simulink model "AMCLIB_BemfObsrvDQ_BAM"  (Simulink 9.3)
settings: Solver=VariableStepAuto  StartTime=0.0  StopTime=10.0  RelTol=1e-3
settings Model: Creator=nxa18952  LastModifiedBy=nxa18952
settings DataIOCC: SaveFormat=Dataset  SignalLoggingSaveFormat=Dataset  ReturnWorkspaceOutputs=on
settings OptimizationCC: LifeSpan=auto
settings DebuggingCC: UnderspecifiedInitializationDetection=Simplified  MergeDetectMultiDrivingBlocksExec=error  FcnCallInpInsideContextMsg=error  SFUnexpectedBacktrackingDiag=error  SFNoUnconditionalDefaultTransitionDiag=error  SFExecutionAtInitializationDiag=warning  ArithmeticOperatorsInVariantConditions=error
settings HardwareCC: ProdBitPerPointer=64  ProdBitPerSizeT=64  ProdBitPerPtrDiffT=64  ProdLargestAtomicFloat=Float  ProdIntDivRoundTo=Zero  ProdEndianess=LittleEndian  ProdWordSize=64  ProdHWDeviceType=Intel->x86-64 (Windows64)
settings ModelReferenceCC: PropagateSignalLabelsOutOfModel=on
settings SFSimCC: SimUseLocalCustomCode=on
settings RTWCC: RTWUseLocalCustomCode=on
settings CodeAppCC: StateflowObjectComments=off
settings GRTTargetCC: TargetLangStandard=C99 (ISO)  CombineOutputUpdateFcns=on  GRTInterface=off
settings ConfigComp: CovMetricSettings=dwe  CovHtmlReporting=off  CovSaveCumulativeToWorkspaceVar=off  CovSaveSingleToWorkspaceVar=off  CovExternalEMLEnable=on

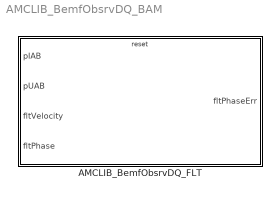
== system AMCLIB_BemfObsrvDQ_BAM ==
  AMCLIB_BemfObsrvDQ_FLT : Subsystem  TreatAsAtomicUnit=on  mask(AMCLIB_BemfObsrvDQ_FLT){showStates=Hide (faster execution), resetStatesEnable=Pre-set according to the first set of inputs after reset, fltIGain=0, fltUGain=0, fltWIGain=0, fltEGain=0, fltCC1sc_D=0, fltCC2sc_D=0, fltUpperLimit_D=0, fltLowerLimit_D=0, fltCC1sc_Q=0, fltCC2sc_Q=0, fltUpperLimit_Q=0, fltLowerLimit_Q=0}
      mask prompts: showStates "Show internal states"; resetStatesEnable "Internal state after reset"; fltIGain "fltIGain (RL circuit constant)"; fltUGain "fltUGain (Voltage cross-coupling constant)"; fltWIGain "fltWIGain (Angular velocity cross-coupling constant)"; fltEGain "fltEGain (Back-EMF cross-coupling constant)"; fltCC1sc_D "fltCC1sc_D (CC1 coefficient of the D-axis PI controller)"; fltCC2sc_D "fltCC2sc_D (CC2 coefficient of the D-axis PI controller)"; fltUpperLimit_D "fltUpperLimit_D (Upper Limit of the D-axis PI controller)"; fltLowerLimit_D "fltLowerLimit_D (Lower Limit of the D-axis PI controller)"; fltCC1sc_Q "fltCC1sc_Q (CC1 coefficient of the Q-axis PI controller)"; fltCC2sc_Q "fltCC2sc_Q (CC2 coefficient of the Q-axis PI controller)"; fltUpperLimit_Q "fltUpperLimit_Q (Upper Limit of the Q-axis PI controller)"; fltLowerLimit_Q "fltLowerLimit_Q (Lower Limit of the Q-axis PI controller)"
      mask help: PMSM back-EMF observer DQ in single precision floating-point implementation. This block supports re-initialization of the internal state during simulation. If the block is reset, the observer will align with the motor's position and speed measured in the next time step. This allows seamless on-the-fly transition to the closed-loop control. Refer to the AMMCLIB User's Guide for further details.
      mask init:
      | if ~evalin('base','exist(''tS8'',''var'')')
      |   if (2 ~= exist('SWLIBS_Typedefs.mat','file'))
      |       error('File SWLIBS_Typedefs.mat is not on the Matlab path. Please add the AMMCLIB "bam" folder in the Matlab Search Path.');
      |   else
      |       evalin('base', 'load(''SWLIBS_Typedefs.mat'')');
      |   end
      | end
      | if showStates == 1
      |     % hidden state variables
      |     if strcmp(get_param([gcb '/fltIGain'], 'BlockType'), 'Inport')
      |         posblk = get_param(gcb, 'Position');
      | 
      |         pos = get_param(    [gcb, '/fltIGain'], 'Position');
      |         orient = get_param( [gcb, '/fltIGain'], 'Orientation');
      |         delete_block(       [gcb, '/fltIGain']);
      |         add_block('built-in/Ground', [gcb, '/fltIGain'], 'Position', pos, 'Orientation', orient);
      | 
      |         pos = get_param(    [gcb, '/fltUGain'], 'Position');
      |         orient = get_param( [gcb, '/fltUGain'], 'Orientation');
      |         delete_block(       [gcb, '/fltUGain']);
      |         add_block('built-in/Ground', [gcb, '/fltUGain'], 'Position', pos, 'Orientation', orient);
      | 
      |         pos = get_param(    [gcb, '/fltWIGain'], 'Position');
      |         orient = get_param( [gcb, '/fltWIGain'], 'Orientation');
      |         delete_block(       [gcb, '/fltWIGain']);
      |         add_block('built-in/Ground', [gcb, '/fltWIGain'], 'Position', pos, 'Orientation', orient);
      | 
      |         pos = get_param(    [gcb, '/fltEGain'], 'Position');
      |         orient = get_param( [gcb, '/fltEGain'], 'Orientation');
      |         delete_block(       [gcb, '/fltEGain']);
      |         add_block('built-in/Ground', [gcb, '/fltEGain'], 'Position', pos, 'Orientation', orient);
      | 
      |         pos = get_param(    [gcb, '/fltCC1sc_D'], 'Position');
      |         orient = get_param( [gcb, '/fltCC1sc_D'], 'Orientation');
      |         delete_block(       [gcb, '/fltCC1sc_D']);
      |         add_block('built-in/Ground', [gcb, '/fltCC1sc_D'], 'Position', pos, 'Orientation', orient);
      | 
      |         pos = get_param(    [gcb, '/fltCC2sc_D'], 'Position');
      |         orient = get_param( [gcb, '/fltCC2sc_D'], 'Orientation');
      |         delete_block(       [gcb, '/fltCC2sc_D']);
      |         add_block('built-in/Ground', [gcb, '/fltCC2sc_D'], 'Position', pos, 'Orientation', orient);
      | 
      |         pos = get_param(    [gcb, '/fltUpperLimit_D'], 'Position');
      |         orient = get_param( [gcb, '/fltUpperLimit_D'], 'Orientation');
      |         delete_block(       [gcb, '/fltUpperLimit_D']);
      |         add_block('built-in/Ground', [gcb, '/fltUpperLimit_D'], 'Position', pos, 'Orientation', orient);
      | 
      |         pos = get_param(    [gcb, '/fltLowerLimit_D'], 'Position');
      |         orient = get_param( [gcb, '/fltLowerLimit_D'], 'Orientation');
      |         delete_block(       [gcb, '/fltLowerLimit_D']);
      |         add_block('built-in/Ground', [gcb, '/fltLowerLimit_D'], 'Position', pos, 'Orientation', orient);
      | 
      |         pos = get_param(    [gcb, '/fltCC1sc_Q'], 'Position');
      |         orient = get_param( [gcb, '/fltCC1sc_Q'], 'Orientation');
      |         delete_block(       [gcb, '/fltCC1sc_Q']);
      |         add_block('built-in/Ground', [gcb, '/fltCC1sc_Q'], 'Position', pos, 'Orientation', orient);
      | 
      |         pos = get_param(    [gcb, '/fltCC2sc_Q'], 'Position');
      |         orient = get_param( [gcb, '/fltCC2sc_Q'], 'Orientation');
      |         delete_block(       [gcb, '/fltCC2sc_Q']);
      |         add_block('built-in/Ground', [gcb, '/fltCC2sc_Q'], 'Position', pos, 'Orientation', orient);
      | 
      |         pos = get_param(    [gcb, '/fltUpperLimit_Q'], 'Position');
      |         orient = get_param( [gcb, '/fltUpperLimit_Q'], 'Orientation');
      |         delete_block(       [gcb, '/fltUpperLimit_Q']);
      |         add_block('built-in/Ground', [gcb, '/fltUpperLimit_Q'], 'Position', pos, 'Orientation', orient);
      | 
      |         pos = get_param(    [gcb, '/fltLowerLimit_Q'], 'Position');
      |         orient = get_param( [gcb, '/fltLowerLimit_Q'], 'Orientation');
      |         delete_block(       [gcb, '/fltLowerLimit_Q']);
      |         add_block('built-in/Ground', [gcb, '/fltLowerLimit_Q'], 'Position', pos, 'Orientation', orient);
      | 
      |         pos = get_param(    [gcb, '/fltAcc_D'], 'Position');
      |         orient = get_param( [gcb, '/fltAcc_D'], 'Orientation');
      |         delete_block(       [gcb, '/fltAcc_D']);
      |         add_block('built-in/Ground', [gcb, '/fltAcc_D'], 'Position', pos, 'Orientation', orient);
      | 
      |         pos = get_param(    [gcb, '/fltInErrK1_D'], 'Position');
      |         orient = get_param( [gcb, '/fltInErrK1_D'], 'Orientation');
      |         delete_block(       [gcb, '/fltInErrK1_D']);
      |         add_block('built-in/Ground', [gcb, '/fltInErrK1_D'], 'Position', pos, 'Orientation', orient);
      | 
      |         pos = get_param(    [gcb, '/fltAcc_Q'], 'Position');
      |         orient = get_param( [gcb, '/fltAcc_Q'], 'Orientation');
      |         delete_block(       [gcb, '/fltAcc_Q']);
      |         add_block('built-in/Ground', [gcb, '/fltAcc_Q'], 'Position', pos, 'Orientation', orient);
      | 
      |         pos = get_param(    [gcb, '/fltInErrK1_Q'], 'Position');
      |         orient = get_param( [gcb, '/fltInErrK1_Q'], 'Orientation');
      |         delete_block(       [gcb, '/fltInErrK1_Q']);
      |         add_block('built-in/Ground', [gcb, '/fltInErrK1_Q'], 'Position', pos, 'Orientation', orient);
      | 
      |         pos = get_param(    [gcb, '/fltIObsrvIn_1_D'], 'Position');
      |         orient = get_param( [gcb, '/fltIObsrvIn_1_D'], 'Orientation');
      |         delete_block(       [gcb, '/fltIObsrvIn_1_D']);
      |         add_block('built-in/Ground', [gcb, '/fltIObsrvIn_1_D'], 'Position', pos, 'Orientation', orient);
      | 
      |         pos = get_param(    [gcb, '/fltIObsrvIn_1_Q'], 'Position');
      |         orient = get_param( [gcb, '/fltIObsrvIn_1_Q'], 'Orientation');
      |         delete_block(       [gcb, '/fltIObsrvIn_1_Q']);
      |         add_block('built-in/Ground', [gcb, '/fltIObsrvIn_1_Q'], 'Position', pos, 'Orientation', orient);
      | 
      |         pos = get_param(    [gcb, '/fltIObsrv_D'], 'Position');
      |         orient = get_param( [gcb, '/fltIObsrv_D'], 'Orientation');
      |         delete_block(       [gcb, '/fltIObsrv_D']);
      |         add_block('built-in/Ground', [gcb, '/fltIObsrv_D'], 'Position', pos, 'Orientation', orient);
      | 
      |         pos = get_param(    [gcb, '/fltIObsrv_Q'], 'Position');
      |         orient = get_param( [gcb, '/fltIObsrv_Q'], 'Orientation');
      |         delete_block(       [gcb, '/fltIObsrv_Q']);
      |         add_block('built-in/Ground', [gcb, '/fltIObsrv_Q'], 'Position', pos, 'Orientation', orient);
      | 
      | 
      |         pos = get_param(    [gcb '/fltEObsrv_D_Out'], 'Position');
      |         orient = get_param( [gcb '/fltEObsrv_D_Out'], 'Orientation');
      |         delete_block(       [gcb '/fltEObsrv_D_Out']);
      |         add_block('built-in/Terminator', [gcb '/fltEObsrv_D_Out'], 'Position', pos, 'Orientation', orient);
      | 
      |         pos = get_param(    [gcb '/fltEObsrv_Q_Out'], 'Position');
      |         orient = get_param( [gcb '/fltEObsrv_Q_Out'], 'Orientation');
      |         delete_block(       [gcb '/fltEObsrv_Q_Out']);
      |         add_block('built-in/Terminator', [gcb '/fltEObsrv_Q_Out'], 'Position', pos, 'Orientation', orient);
      | 
      |         pos = get_param(    [gcb '/fltAcc_D_Out'], 'Position');
      |         orient = get_param( [gcb '/fltAcc_D_Out'], 'Orientation');
      |         delete_block(       [gcb '/fltAcc_D_Out']);
      |         add_block('built-in/Terminator', [gcb '/fltAcc_D_Out'], 'Position', pos, 'Orientation', orient);
      | 
      |         pos = get_param(    [gcb '/fltInErrK1_D_Out'], 'Position');
      |         orient = get_param( [gcb '/fltInErrK1_D_Out'], 'Orientation');
      |         delete_block(       [gcb '/fltInErrK1_D_Out']);
      |         add_block('built-in/Terminator', [gcb '/fltInErrK1_D_Out'], 'Position', pos, 'Orientation', orient);
      | 
      |         pos = get_param(    [gcb '/fltAcc_Q_Out'], 'Position');
      |         orient = get_param( [gcb '/fltAcc_Q_Out'], 'Orientation');
      |         delete_block(       [gcb '/fltAcc_Q_Out']);
      |         add_block('built-in/Terminator', [gcb '/fltAcc_Q_Out'], 'Position', pos, 'Orientation', orient);
      | 
      |         pos = get_param(    [gcb '/fltInErrK1_Q_Out'], 'Position');
      |         orient = get_param( [gcb '/fltInErrK1_Q_Out'], 'Orientation');
      |         delete_block(       [gcb '/fltInErrK1_Q_Out']);
      |         add_block('built-in/Terminator', [gcb '/fltInErrK1_Q_Out'], 'Position', pos, 'Orientation', orient);
      | 
      |         pos = get_param(    [gcb '/fltIObsrvIn_1_D_Out'], 'Position');
      |         orient = get_param( [gcb '/fltIObsrvIn_1_D_Out'], 'Orientation');
      |         delete_block(       [gcb '/fltIObsrvIn_1_D_Out']);
      |         add_block('built-in/Terminator', [gcb '/fltIObsrvIn_1_D_Out'], 'Position', pos, 'Orientation', orient);
      | 
      |         pos = get_param(    [gcb '/fltIObsrvIn_1_Q_Out'], 'Position');
      |         orient = get_param( [gcb '/fltIObsrvIn_1_Q_Out'], 'Orientation');
      |         delete_block(       [gcb '/fltIObsrvIn_1_Q_Out']);
      |         add_block('built-in/Terminator', [gcb '/fltIObsrvIn_1_Q_Out'], 'Position', pos, 'Orientation', orient);
      | 
      |         pos = get_param(    [gcb '/fltIObsrv_D_Out'], 'Position');
      |         orient = get_param( [gcb '/fltIObsrv_D_Out'], 'Orientation');
      |         delete_block(       [gcb '/fltIObsrv_D_Out']);
      |         add_block('built-in/Terminator', [gcb '/fltIObsrv_D_Out'], 'Position', pos, 'Orientation', orient);
      | 
      |         pos = get_param(    [gcb '/fltIObsrv_Q_Out'], 'Position');
      |         orient = get_param( [gcb '/fltIObsrv_Q_Out'], 'Orientation');
      |         delete_block(       [gcb '/fltIObsrv_Q_Out']);
      |         add_block('built-in/Terminator', [gcb '/fltIObsrv_Q_Out'], 'Position', pos, 'Orientation', orient);
      | 
      | 
      |         set_param([gcb '/pIAB'], 'Port', '1');
      |         set_param([gcb '/pUAB'], 'Port', '2');
      |         set_param([gcb '/fltVelocity'], 'Port', '3');
      |         set_param([gcb '/fltPhase'], 'Port', '4');
      | 
      |         set_param([gcb '/fltPhaseErr'], 'Port', '1');
      | 
      |         set_param(gcb,'MaskEnables',{'on','on','on','on','on','on','on','on','on','on','on','on','on','on'});
      | 
      |         if (posblk(4) - posblk(2)) > 125
      |           height = 125;
      |           set_param(gcb,'Position',[posblk(1), posblk(2), posblk(3), posblk(2)+height])
      |         end
      |     end
      | else
      |     % shown state variables
      |     if strcmp(get_param([gcb '/fltIGain'], 'BlockType'), 'Ground')
      |         posblk = get_param(gcb, 'Position');
      | 
      |         pos = get_param(    [gcb, '/fltIGain'], 'Position');
      |         orient = get_param( [gcb, '/fltIGain'], 'Orientation');
      |         delete_block(       [gcb, '/fltIGain']);
      |         add_block('built-in/Inport', [gcb, '/fltIGain'], 'Position', pos, 'Orientation', orient, 'OutDataTypeStr', 'single');
      | 
      |         pos = get_param(    [gcb, '/fltUGain'], 'Position');
      |         orient = get_param( [gcb, '/fltUGain'], 'Orientation');
      |         delete_block(       [gcb, '/fltUGain']);
      |         add_block('built-in/Inport', [gcb, '/fltUGain'], 'Position', pos, 'Orientation', orient, 'OutDataTypeStr', 'single');
      | 
      |         pos = get_param(    [gcb, '/fltWIGain'], 'Position');
      |         orient = get_param( [gcb, '/fltWIGain'], 'Orientation');
      |         delete_block(       [gcb, '/fltWIGain']);
      |         add_block('built-in/Inport', [gcb, '/fltWIGain'], 'Position', pos, 'Orientation', orient, 'OutDataTypeStr', 'single');
      | 
      |         pos = get_param(    [gcb, '/fltEGain'], 'Position');
      |         orient = get_param( [gcb, '/fltEGain'], 'Orientation');
      |         delete_block(       [gcb, '/fltEGain']);
      |         add_block('built-in/Inport', [gcb, '/fltEGain'], 'Position', pos, 'Orientation', orient, 'OutDataTypeStr', 'single');
      | 
      |         pos = get_param(    [gcb, '/fltCC1sc_D'], 'Position');
      |         orient = get_param( [gcb, '/fltCC1sc_D'], 'Orientation');
      |         delete_block(       [gcb, '/fltCC1sc_D']);
      |         add_block('built-in/Inport', [gcb, '/fltCC1sc_D'], 'Position', pos, 'Orientation', orient, 'OutDataTypeStr', 'single');
      | 
      |         pos = get_param(    [gcb, '/fltCC2sc_D'], 'Position');
      |         orient = get_param( [gcb, '/fltCC2sc_D'], 'Orientation');
      |         delete_block(       [gcb, '/fltCC2sc_D']);
      |         add_block('built-in/Inport', [gcb, '/fltCC2sc_D'], 'Position', pos, 'Orientation', orient, 'OutDataTypeStr', 'single');
      | 
      |         pos = get_param(    [gcb, '/fltUpperLimit_D'], 'Position');
      |         orient = get_param( [gcb, '/fltUpperLimit_D'], 'Orientation');
      |         delete_block(       [gcb, '/fltUpperLimit_D']);
      |         add_block('built-in/Inport', [gcb, '/fltUpperLimit_D'], 'Position', pos, 'Orientation', orient, 'OutDataTypeStr', 'single');
      | 
      |         pos = get_param(    [gcb, '/fltLowerLimit_D'], 'Position');
      |         orient = get_param( [gcb, '/fltLowerLimit_D'], 'Orientation');
      |         delete_block(       [gcb, '/fltLowerLimit_D']);
      |         add_block('built-in/Inport', [gcb, '/fltLowerLimit_D'], 'Position', pos, 'Orientation', orient, 'OutDataTypeStr', 'single');
      | 
      |         pos = get_param(    [gcb, '/fltCC1sc_Q'], 'Position');
      |         orient = get_param( [gcb, '/fltCC1sc_Q'], 'Orientation');
      |         delete_block(       [gcb, '/fltCC1sc_Q']);
      |         add_block('built-in/Inport', [gcb, '/fltCC1sc_Q'], 'Position', pos, 'Orientation', orient, 'OutDataTypeStr', 'single');
      | 
      |         pos = get_param(    [gcb, '/fltCC2sc_Q'], 'Position');
      |         orient = get_param( [gcb, '/fltCC2sc_Q'], 'Orientation');
      |         delete_block(       [gcb, '/fltCC2sc_Q']);
      |         add_block('built-in/Inport', [gcb, '/fltCC2sc_Q'], 'Position', pos, 'Orientation', orient, 'OutDataTypeStr', 'single');
      | 
      |         pos = get_param(    [gcb, '/fltUpperLimit_Q'], 'Position');
      |         orient = get_param( [gcb, '/fltUpperLimit_Q'], 'Orientation');
      |         delete_block(       [gcb, '/fltUpperLimit_Q']);
      |         add_block('built-in/Inport', [gcb, '/fltUpperLimit_Q'], 'Position', pos, 'Orientation', orient, 'OutDataTypeStr', 'single');
      | 
      |         pos = get_param(    [gcb, '/fltLowerLimit_Q'], 'Position');
      |         orient = get_param( [gcb, '/fltLowerLimit_Q'], 'Orientation');
      |         delete_block(       [gcb, '/fltLowerLimit_Q']);
      |         add_block('built-in/Inport', [gcb, '/fltLowerLimit_Q'], 'Position', pos, 'Orientation', orient, 'OutDataTypeStr', 'single');
      | 
      |         pos = get_param(    [gcb, '/fltAcc_D'], 'Position');
      |         orient = get_param( [gcb, '/fltAcc_D'], 'Orientation');
      |         delete_block(       [gcb, '/fltAcc_D']);
      |         add_block('built-in/Inport', [gcb, '/fltAcc_D'], 'Position', pos, 'Orientation', orient, 'OutDataTypeStr', 'single');
      | 
      |         pos = get_param(    [gcb, '/fltInErrK1_D'], 'Position');
      |         orient = get_param( [gcb, '/fltInErrK1_D'], 'Orientation');
      |         delete_block(       [gcb, '/fltInErrK1_D']);
      |         add_block('built-in/Inport', [gcb, '/fltInErrK1_D'], 'Position', pos, 'Orientation', orient, 'OutDataTypeStr', 'single');
      | 
      |         pos = get_param(    [gcb, '/fltAcc_Q'], 'Position');
      |         orient = get_param( [gcb, '/fltAcc_Q'], 'Orientation');
      |         delete_block(       [gcb, '/fltAcc_Q']);
      |         add_block('built-in/Inport', [gcb, '/fltAcc_Q'], 'Position', pos, 'Orientation', orient, 'OutDataTypeStr', 'single');
      | 
      |         pos = get_param(    [gcb, '/fltInErrK1_Q'], 'Position');
      |         orient = get_param( [gcb, '/fltInErrK1_Q'], 'Orientation');
      |         delete_block(       [gcb, '/fltInErrK1_Q']);
      |         add_block('built-in/Inport', [gcb, '/fltInErrK1_Q'], 'Position', pos, 'Orientation', orient, 'OutDataTypeStr', 'single');
      | 
      |         pos = get_param(    [gcb, '/fltIObsrvIn_1_D'], 'Position');
      |         orient = get_param( [gcb, '/fltIObsrvIn_1_D'], 'Orientation');
      |         delete_block(       [gcb, '/fltIObsrvIn_1_D']);
      |         add_block('built-in/Inport', [gcb, '/fltIObsrvIn_1_D'], 'Position', pos, 'Orientation', orient, 'OutDataTypeStr', 'single');
      | 
      |         pos = get_param(    [gcb, '/fltIObsrvIn_1_Q'], 'Position');
      |         orient = get_param( [gcb, '/fltIObsrvIn_1_Q'], 'Orientation');
      |         delete_block(       [gcb, '/fltIObsrvIn_1_Q']);
      |         add_block('built-in/Inport', [gcb, '/fltIObsrvIn_1_Q'], 'Position', pos, 'Orientation', orient, 'OutDataTypeStr', 'single');
      | 
      |         pos = get_param(    [gcb, '/fltIObsrv_D'], 'Position');
      |         orient = get_param( [gcb, '/fltIObsrv_D'], 'Orientation');
      |         delete_block(       [gcb, '/fltIObsrv_D']);
      |         add_block('built-in/Inport', [gcb, '/fltIObsrv_D'], 'Position', pos, 'Orientation', orient, 'OutDataTypeStr', 'single');
      | 
      |         pos = get_param(    [gcb, '/fltIObsrv_Q'], 'Position');
      |         orient = get_param( [gcb, '/fltIObsrv_Q'], 'Orientation');
      |         delete_block(       [gcb, '/fltIObsrv_Q']);
      |         add_block('built-in/Inport', [gcb, '/fltIObsrv_Q'], 'Position', pos, 'Orientation', orient, 'OutDataTypeStr', 'single');
      | 
      | 
      |         pos = get_param(    [gcb '/fltEObsrv_D_Out'], 'Position');
      |         orient = get_param( [gcb '/fltEObsrv_D_Out'], 'Orientation');
      |         delete_block(       [gcb '/fltEObsrv_D_Out']);
      |         add_block('built-in/Outport', [gcb '/fltEObsrv_D_Out'], 'Position', pos, 'Orientation', orient);
      | 
      |         pos = get_param(    [gcb '/fltEObsrv_Q_Out'], 'Position');
      |         orient = get_param( [gcb '/fltEObsrv_Q_Out'], 'Orientation');
      |         delete_block(       [gcb '/fltEObsrv_Q_Out']);
      |         add_block('built-in/Outport', [gcb '/fltEObsrv_Q_Out'], 'Position', pos, 'Orientation', orient);
      | 
      |         pos = get_param(    [gcb '/fltAcc_D_Out'], 'Position');
      |         orient = get_param( [gcb '/fltAcc_D_Out'], 'Orientation');
      |         delete_block(       [gcb '/fltAcc_D_Out']);
      |         add_block('built-in/Outport', [gcb '/fltAcc_D_Out'], 'Position', pos, 'Orientation', orient);
      | 
      |         pos = get_param(    [gcb '/fltInErrK1_D_Out'], 'Position');
      |         orient = get_param( [gcb '/fltInErrK1_D_Out'], 'Orientation');
      |         delete_block(       [gcb '/fltInErrK1_D_Out']);
      |         add_block('built-in/Outport', [gcb '/fltInErrK1_D_Out'], 'Position', pos, 'Orientation', orient);
      | 
      |         pos = get_param(    [gcb '/fltAcc_Q_Out'], 'Position');
      |         orient = get_param( [gcb '/fltAcc_Q_Out'], 'Orientation');
      |         delete_block(       [gcb '/fltAcc_Q_Out']);
      |         add_block('built-in/Outport', [gcb '/fltAcc_Q_Out'], 'Position', pos, 'Orientation', orient);
      | 
      |         pos = get_param(    [gcb '/fltInErrK1_Q_Out'], 'Position');
      |         orient = get_param( [gcb '/fltInErrK1_Q_Out'], 'Orientation');
      |         delete_block(       [gcb '/fltInErrK1_Q_Out']);
      |         add_block('built-in/Outport', [gcb '/fltInErrK1_Q_Out'], 'Position', pos, 'Orientation', orient);
      | 
      |         pos = get_param(    [gcb '/fltIObsrvIn_1_D_Out'], 'Position');
      |         orient = get_param( [gcb '/fltIObsrvIn_1_D_Out'], 'Orientation');
      |         delete_block(       [gcb '/fltIObsrvIn_1_D_Out']);
      |         add_block('built-in/Outport', [gcb '/fltIObsrvIn_1_D_Out'], 'Position', pos, 'Orientation', orient);
      | 
      |         pos = get_param(    [gcb '/fltIObsrvIn_1_Q_Out'], 'Position');
      |         orient = get_param( [gcb '/fltIObsrvIn_1_Q_Out'], 'Orientation');
      |         delete_block(       [gcb '/fltIObsrvIn_1_Q_Out']);
      |         add_block('built-in/Outport', [gcb '/fltIObsrvIn_1_Q_Out'], 'Position', pos, 'Orientation', orient);
      | 
      |         pos = get_param(    [gcb '/fltIObsrv_D_Out'], 'Position');
      |         orient = get_param( [gcb '/fltIObsrv_D_Out'], 'Orientation');
      |         delete_block(       [gcb '/fltIObsrv_D_Out']);
      |         add_block('built-in/Outport', [gcb '/fltIObsrv_D_Out'], 'Position', pos, 'Orientation', orient);
      | 
      |         pos = get_param(    [gcb '/fltIObsrv_Q_Out'], 'Position');
      |         orient = get_param( [gcb '/fltIObsrv_Q_Out'], 'Orientation');
      |         delete_block(       [gcb '/fltIObsrv_Q_Out']);
      |         add_block('built-in/Outport', [gcb '/fltIObsrv_Q_Out'], 'Position', pos, 'Orientation', orient);
      | 
      | 
      |         set_param([gcb '/pIAB'], 'Port', '1');
      |         set_param([gcb '/pUAB'], 'Port', '2');
      |         set_param([gcb '/fltVelocity'], 'Port', '3');
      |         set_param([gcb '/fltPhase'], 'Port', '4');
      |         set_param([gcb '/fltIGain'], 'Port', '5');
      |         set_param([gcb '/fltUGain'], 'Port', '6');
      |         set_param([gcb '/fltWIGain'], 'Port', '7');
      |         set_param([gcb '/fltEGain'], 'Port', '8');
      |         set_param([gcb '/fltCC1sc_D'], 'Port', '9');
      |         set_param([gcb '/fltCC2sc_D'], 'Port', '10');
      |         set_param([gcb '/fltUpperLimit_D'], 'Port', '11');
      |         set_param([gcb '/fltLowerLimit_D'], 'Port', '12');
      |         set_param([gcb '/fltCC1sc_Q'], 'Port', '13');
      |         set_param([gcb '/fltCC2sc_Q'], 'Port', '14');
      |         set_param([gcb '/fltUpperLimit_Q'], 'Port', '15');
      |         set_param([gcb '/fltLowerLimit_Q'], 'Port', '16');
      |         set_param([gcb '/fltAcc_D'], 'Port', '17');
      |         set_param([gcb '/fltInErrK1_D'], 'Port', '18');
      |         set_param([gcb '/fltAcc_Q'], 'Port', '19');
      |         set_param([gcb '/fltInErrK1_Q'], 'Port', '20');
      |         set_param([gcb '/fltIObsrvIn_1_D'], 'Port', '21');
      |         set_param([gcb '/fltIObsrvIn_1_Q'], 'Port', '22');
      |         set_param([gcb '/fltIObsrv_D'], 'Port', '23');
      |         set_param([gcb '/fltIObsrv_Q'], 'Port', '24');
      | 
      |         set_param([gcb '/fltPhaseErr'], 'Port', '1');
      |         set_param([gcb '/fltEObsrv_D_Out'], 'Port', '2');
      |         set_param([gcb '/fltEObsrv_Q_Out'], 'Port', '3');
      |         set_param([gcb '/fltAcc_D_Out'], 'Port', '4');
      |         set_param([gcb '/fltInErrK1_D_Out'], 'Port', '5');
      |         set_param([gcb '/fltAcc_Q_Out'], 'Port', '6');
      |         set_param([gcb '/fltInErrK1_Q_Out'], 'Port', '7');
      |         set_param([gcb '/fltIObsrvIn_1_D_Out'], 'Port', '8');
      |         set_param([gcb '/fltIObsrvIn_1_Q_Out'], 'Port', '9');
      |         set_param([gcb '/fltIObsrv_D_Out'], 'Port', '10');
      |         set_param([gcb '/fltIObsrv_Q_Out'], 'Port', '11');
      | 
      |         set_param(gcb,'MaskEnables',{'on','on','off','off','off','off','off','off','off','off','off','off','off','off'});
      | 
      |         if (posblk(4) - posblk(2)) < 625
      |           height = 625;
      |           set_param(gcb,'Position',[posblk(1), posblk(2), posblk(3), posblk(2)+height])
      |         end
      |     end
      | end
      settings: RTWSystemCode=Inline
      mask TypeOptions showStates: Hide (faster execution) | Show (allows debugging; connect feedback loops manually)
      mask Callback showStates:
      | maskStr = get_param(gcb,'showStates');
      | if strcmp(maskStr,'Hide (faster execution)'),
      |     set_param(gcb,'MaskEnables',{'on','on','on','on','on','on','on','on','on','on','on','on','on','on'});
      | else
      |     set_param(gcb,'MaskEnables',{'on','on','off','off','off','off','off','off','off','off','off','off','off','off'});
      | end
      mask TypeOptions resetStatesEnable: Pre-set according to the first set of inputs after reset | Clear to zero
      mask Display:
      | color('black');
      | pos = get_param(gcb, 'Position');
      | width = pos(3) - pos(1);
      | height = pos(4) - pos(2);
      | tX=width/2;
      | tY=height - 25;
      | color('black');
      | text(tX,tY, 'AMCLIB_BemfObsrvDQ_FLT', 'horizontalAlignment', 'center');
      | if showStates == 2
      |   color('red');
      |   text(tX,tY - 20, ['debugging mode' char(13) char(10) '(limited performance)'], 'horizontalAlignment', 'center');
      | end

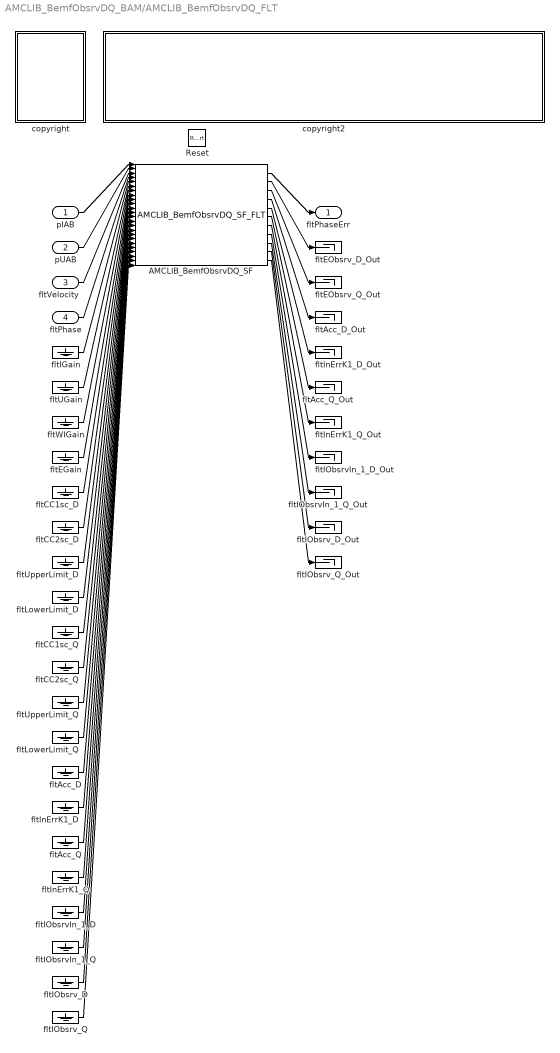
== system AMCLIB_BemfObsrvDQ_BAM/AMCLIB_BemfObsrvDQ_FLT ==
  pIAB : Inport  OutDataTypeStr=Bus: SWLIBS_2Syst_FLT  BusOutputAsStruct=on
  pUAB : Inport  Port=2  OutDataTypeStr=Bus: SWLIBS_2Syst_FLT  BusOutputAsStruct=on
  fltVelocity : Inport  Port=3  OutDataTypeStr=single
  fltPhase : Inport  Port=4  OutDataTypeStr=single
  Reset : ResetPort  DisableCoverage=on
  AMCLIB_BemfObsrvDQ_SF : S-Function  FunctionName=AMCLIB_BemfObsrvDQ_SF_FLT  Parameters=showStates,resetStatesEnable,fltIGain,fltUGain,fltWIGain,fltEGain,fltCC1sc_D,fltCC2sc_D,fltUpperLimit_D,fltLowerLimit_D,fltCC1sc_Q,fltCC2sc_Q,fltUpperLimit_Q,fltLowerLimit_Q  SFunctionDeploymentMode=off  EnableBusSupport=off
  copyright : Subsystem
      mask Display: text(10,90,'FILE:');text(10,75,'DESRIPTION:');text(10,60,'COPYRIGHT:');text(10,45,'VERSION:');text(10,30,'DATE:')
  copyright2 : Subsystem
      mask Display: text(10,90,'AMCLIB_BemfObsrvDQ_BAM_FLT.mdl');text(10,75,'PMSM back-EMF observer DQ.');text(10,60,'NXP 2020');text(10,45,'1.0');text(10,30,'28-Mar-2020');
  fltAcc_D : Ground
  fltAcc_D_Out : Terminator
  fltAcc_Q : Ground
  fltAcc_Q_Out : Terminator
  fltCC1sc_D : Ground
  fltCC1sc_Q : Ground
  fltCC2sc_D : Ground
  fltCC2sc_Q : Ground
  fltEGain : Ground
  fltEObsrv_D_Out : Terminator
  fltEObsrv_Q_Out : Terminator
  fltIGain : Ground
  fltIObsrvIn_1_D : Ground
  fltIObsrvIn_1_D_Out : Terminator
  fltIObsrvIn_1_Q : Ground
  fltIObsrvIn_1_Q_Out : Terminator
  fltIObsrv_D : Ground
  fltIObsrv_D_Out : Terminator
  fltIObsrv_Q : Ground
  fltIObsrv_Q_Out : Terminator
  fltInErrK1_D : Ground
  fltInErrK1_D_Out : Terminator
  fltInErrK1_Q : Ground
  fltInErrK1_Q_Out : Terminator
  fltLowerLimit_D : Ground
  fltLowerLimit_Q : Ground
  fltUGain : Ground
  fltUpperLimit_D : Ground
  fltUpperLimit_Q : Ground
  fltWIGain : Ground
  fltPhaseErr : Outport
  wires:
  pIAB/1 -> AMCLIB_BemfObsrvDQ_SF/1
  pUAB/1 -> AMCLIB_BemfObsrvDQ_SF/2
  fltVelocity/1 -> AMCLIB_BemfObsrvDQ_SF/3
  fltPhase/1 -> AMCLIB_BemfObsrvDQ_SF/4
  fltIGain/1 -> AMCLIB_BemfObsrvDQ_SF/5
  fltUGain/1 -> AMCLIB_BemfObsrvDQ_SF/6
  fltWIGain/1 -> AMCLIB_BemfObsrvDQ_SF/7
  fltEGain/1 -> AMCLIB_BemfObsrvDQ_SF/8
  fltCC1sc_D/1 -> AMCLIB_BemfObsrvDQ_SF/9
  fltCC2sc_D/1 -> AMCLIB_BemfObsrvDQ_SF/10
  fltUpperLimit_D/1 -> AMCLIB_BemfObsrvDQ_SF/11
  fltLowerLimit_D/1 -> AMCLIB_BemfObsrvDQ_SF/12
  fltCC1sc_Q/1 -> AMCLIB_BemfObsrvDQ_SF/13
  fltCC2sc_Q/1 -> AMCLIB_BemfObsrvDQ_SF/14
  fltUpperLimit_Q/1 -> AMCLIB_BemfObsrvDQ_SF/15
  fltLowerLimit_Q/1 -> AMCLIB_BemfObsrvDQ_SF/16
  fltAcc_D/1 -> AMCLIB_BemfObsrvDQ_SF/17
  fltInErrK1_D/1 -> AMCLIB_BemfObsrvDQ_SF/18
  fltAcc_Q/1 -> AMCLIB_BemfObsrvDQ_SF/19
  fltInErrK1_Q/1 -> AMCLIB_BemfObsrvDQ_SF/20
  fltIObsrvIn_1_D/1 -> AMCLIB_BemfObsrvDQ_SF/21
  fltIObsrvIn_1_Q/1 -> AMCLIB_BemfObsrvDQ_SF/22
  fltIObsrv_D/1 -> AMCLIB_BemfObsrvDQ_SF/23
  fltIObsrv_Q/1 -> AMCLIB_BemfObsrvDQ_SF/24
  AMCLIB_BemfObsrvDQ_SF/1 -> fltPhaseErr/1
  AMCLIB_BemfObsrvDQ_SF/2 -> fltEObsrv_D_Out/1
  AMCLIB_BemfObsrvDQ_SF/3 -> fltEObsrv_Q_Out/1
  AMCLIB_BemfObsrvDQ_SF/4 -> fltAcc_D_Out/1
  AMCLIB_BemfObsrvDQ_SF/5 -> fltInErrK1_D_Out/1
  AMCLIB_BemfObsrvDQ_SF/6 -> fltAcc_Q_Out/1
  AMCLIB_BemfObsrvDQ_SF/7 -> fltInErrK1_Q_Out/1
  AMCLIB_BemfObsrvDQ_SF/8 -> fltIObsrvIn_1_D_Out/1
  AMCLIB_BemfObsrvDQ_SF/9 -> fltIObsrvIn_1_Q_Out/1
  AMCLIB_BemfObsrvDQ_SF/10 -> fltIObsrv_D_Out/1
  AMCLIB_BemfObsrvDQ_SF/11 -> fltIObsrv_Q_Out/1

== system AMCLIB_BemfObsrvDQ_BAM/AMCLIB_BemfObsrvDQ_FLT/copyright ==

== system AMCLIB_BemfObsrvDQ_BAM/AMCLIB_BemfObsrvDQ_FLT/copyright2 ==
